simulink model "SimPrac11_2"  (R2018a)
settings: Solver=VariableStepAuto  StartTime=0.0  StopTime=20.0  RelTol=1e-3
values from neighbouring files (symbols this model uses):
  As = [-Ra/La -Kf/La 0 0 -Kusil*Rng/La;   Kf/J 0 0 0 0;   0 1 0 0 0;   0 0 Kr*Ku/Lfg -Rfg/Lfg 0;   0 0 0 Kwg/Lag -(Rag+Rng)/Lag]    [Prac11.m]
  Bs = [ Kusil/La 0 0;   0 -1/J 0;   0 0 0;   0 0 0;   0 0 -1/Lag]    [Prac11.m]
  Cs = [ 0 0 0 0 Rng]    [Prac11.m]
  M = Kf*In    (= 0.0115508291498)    [Prac11.m]
  Ung = 110    [Prac11.m]
settings Model: Creator=dirlak  LastModifiedBy=dirlak

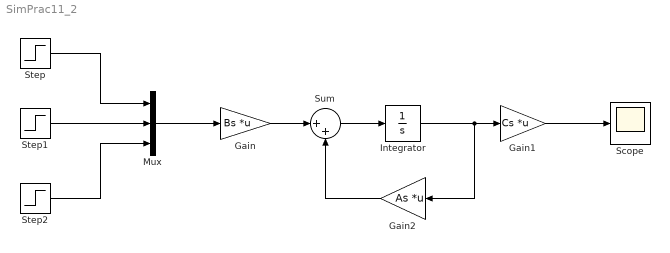
== system SimPrac11_2 ==
  Gain : Gain  Gain=Bs  Multiplication=Matrix(K*u)
  Gain1 : Gain  Gain=Cs  Multiplication=Matrix(K*u)
  Gain2 : Gain  Gain=As  Multiplication=Matrix(K*u)
  Integrator : Integrator
  Mux : Mux  Inputs=3
  Scope : Scope
  Step : Step  Time=0  After=Ung  SampleTime=0
  Step1 : Step  Time=0  After=M  SampleTime=0
  Step2 : Step  Time=10  After=Ung*0.5  SampleTime=0
  Sum : Sum  Inputs=|++
  wires:
  Step/1 -> Mux/1
  Step1/1 -> Mux/2
  Step2/1 -> Mux/3
  Mux/1 -> Gain/1
  Gain/1 -> Sum/1
  Sum/1 -> Integrator/1
  Integrator/1 -> Gain2/1, Gain1/1
  Gain1/1 -> Scope/1
  Gain2/1 -> Sum/2
